simulink model "Pedal_Interpretation_exe"  (Simulink 7.0)
settings: Solver=ode4  StartTime=0.0  StopTime=88  FixedStep=0.01  RelTol=1e-3
InitFcn:
  | PedalInterp_para
values from neighbouring files (symbols this model uses):
  ped_min = 5    [PedalInterp_para.m]
  T_max_Brake = 4000    [PedalInterp_para.m]
  TI = 0    [PAS_callback.m]
undefined symbols (not defined in the file or in its folder): fzgbib, m_ab_100pro, m_ab_70pro, PedalInterpretation, v_bereich
libraries: simulink x320
(part 2 of 23)

== system Pedal_Interpretation_exe/TestData 1/SR-PI-02.2 Acceleration pedal interpretation/Initialisation & Stabilisation ==
  Constant 1 : Constant  Value=0  OutDataType=sfix(16)  OutScaling=2^0
  Constant 2 : Constant  Value=0  OutDataType=sfix(16)  OutScaling=2^0
  Constant 3 : Constant  Value=0  OutDataType=sfix(16)  OutScaling=2^0
  v_Fzg neutral : Outport  OutDataType=sfix(16)  OutScaling=2^0
  phi_Acc neutral : Outport  Port=2  OutDataType=sfix(16)  OutScaling=2^0
  phi_Brake neutral : Outport  Port=3  OutDataType=sfix(16)  OutScaling=2^0
  wires:
  Constant 1/1 -> v_Fzg neutral/1  "Constant 1"
  Constant 2/1 -> phi_Acc neutral/1  "Constant 2"
  Constant 3/1 -> phi_Brake neutral/1  "Constant 3"

== system Pedal_Interpretation_exe/TestData 1/SR-PI-02.2 Acceleration pedal interpretation/v = const & phi_Acc = const ==
  Generate constant 5 : Subsystem
  Generate constant 6 : Subsystem
  v_Fzg : Outport  OutDataType=sfix(16)  OutScaling=2^0
  phi_Acc : Outport  Port=2  OutDataType=sfix(16)  OutScaling=2^0
  wires:
  Generate constant 5/1(v_Fzg) -> v_Fzg/1
  Generate constant 6/1(phi_Acc) -> phi_Acc/1

== system Pedal_Interpretation_exe/TestData 1/SR-PI-02.2 Acceleration pedal interpretation/v = const & phi_Acc decreases & T_des_Drive < 0 ==
  Out Bus : Inport  OutDataType=sfix(16)  OutScaling=2^0
  <Constant>2 : Constant  Value=0  OutDataType=sfix(16)  OutScaling=2^0
  Bound Precond2 : Subsystem  mask(Bound){cm=<}
      mask prompts: cm "Comparison method:"
      mask help:
      | Compare a signal with a reference using the specified comparison method.
      |
      | For '==' or '~=' use "Range - Gap"
      mask init:
      | bp = get_param(gcbh,'Parent');
      | bn = get_param(gcbh,'Name');
      | set_param([bp '/' bn '/RelOp'],'Operator',get_param(gcbh,'cm'));
      mask StyleString: popup(>|>=|<=|<)
      mask Display:
      | port_label('output', 1, 'A');
      | port_label('input', 1, 'Sig');
      | port_label('input', 2, 'Ref');
      | text(0.05,0.5,get_param(get_param([get_param(gcb,'Parent') '/' get_param(gcb,'Name') '/RelOp'],'handle'),'Operator'));
  Bus Selector : BusSelector  OutputSignals=signal1.T_des_Drive
  Generate constant 6 : Subsystem
  Generate decrease 7 : Subsystem
  Memory T_des_Drive : Memory
  Activate : Outport  OutDataType=sfix(16)  OutScaling=2^0
  v_Fzg : Outport  Port=2  OutDataType=sfix(16)  OutScaling=2^0
  phi_Acc : Outport  Port=3  OutDataType=sfix(16)  OutScaling=2^0
  wires:
  Out Bus/1 -> Bus Selector/1
  Bus Selector/1 -> Memory T_des_Drive/1  "<T_des_Drive>"
  Memory T_des_Drive/1 -> Bound Precond2/1(Signal)
  <Constant>2/1 -> Bound Precond2/2(Reference)
  Bound Precond2/1(Activate) -> Activate/1
  Generate constant 6/1(v_Fzg) -> v_Fzg/1
  Generate decrease 7/1(phi_Acc) -> phi_Acc/1

== system Pedal_Interpretation_exe/TestData 1/SR-PI-02.2 Acceleration pedal interpretation/v = const & phi_Acc decreases & T_des_Drive >= 0 ==
  Out Bus : Inport  OutDataType=sfix(16)  OutScaling=2^0
  <Constant>2 : Constant  Value=0  OutDataType=sfix(16)  OutScaling=2^0
  Bound Precond2 : Subsystem  mask(Bound){cm=>=}
      mask prompts: cm "Comparison method:"
      mask help:
      | Compare a signal with a reference using the specified comparison method.
      |
      | For '==' or '~=' use "Range - Gap"
      mask init:
      | bp = get_param(gcbh,'Parent');
      | bn = get_param(gcbh,'Name');
      | set_param([bp '/' bn '/RelOp'],'Operator',get_param(gcbh,'cm'));
      mask StyleString: popup(>|>=|<=|<)
      mask Display:
      | port_label('output', 1, 'A');
      | port_label('input', 1, 'Sig');
      | port_label('input', 2, 'Ref');
      | text(0.05,0.5,get_param(get_param([get_param(gcb,'Parent') '/' get_param(gcb,'Name') '/RelOp'],'handle'),'Operator'));
  Bus Selector : BusSelector  OutputSignals=signal1.T_des_Drive
  Generate constant 6 : Subsystem
  Generate decrease 7 : Subsystem
  Memory T_des_Drive : Memory
  Activate : Outport  OutDataType=sfix(16)  OutScaling=2^0
  v_Fzg : Outport  Port=2  OutDataType=sfix(16)  OutScaling=2^0
  phi_Acc : Outport  Port=3  OutDataType=sfix(16)  OutScaling=2^0
  wires:
  Out Bus/1 -> Bus Selector/1
  Bus Selector/1 -> Memory T_des_Drive/1  "<T_des_Drive>"
  Memory T_des_Drive/1 -> Bound Precond2/1(Signal)
  <Constant>2/1 -> Bound Precond2/2(Reference)
  Bound Precond2/1(Activate) -> Activate/1
  Generate constant 6/1(v_Fzg) -> v_Fzg/1
  Generate decrease 7/1(phi_Acc) -> phi_Acc/1

== system Pedal_Interpretation_exe/TestData 1/SR-PI-02.2 Acceleration pedal interpretation/v = const & phi_Acc increases & T_des_Drive < 0 ==
  Out Bus : Inport  OutDataType=sfix(16)  OutScaling=2^0
  <Constant>2 : Constant  Value=0  OutDataType=sfix(16)  OutScaling=2^0
  Bound Precond2 : Subsystem  mask(Bound){cm=<}
      mask prompts: cm "Comparison method:"
      mask help:
      | Compare a signal with a reference using the specified comparison method.
      |
      | For '==' or '~=' use "Range - Gap"
      mask init:
      | bp = get_param(gcbh,'Parent');
      | bn = get_param(gcbh,'Name');
      | set_param([bp '/' bn '/RelOp'],'Operator',get_param(gcbh,'cm'));
      mask StyleString: popup(>|>=|<=|<)
      mask Display:
      | port_label('output', 1, 'A');
      | port_label('input', 1, 'Sig');
      | port_label('input', 2, 'Ref');
      | text(0.05,0.5,get_param(get_param([get_param(gcb,'Parent') '/' get_param(gcb,'Name') '/RelOp'],'handle'),'Operator'));
  Bus Selector : BusSelector  OutputSignals=signal1.T_des_Drive
  Generate constant 6 : Subsystem
  Generate increase 7 : Subsystem
  Memory T_des_Drive : Memory
  Activate : Outport  OutDataType=sfix(16)  OutScaling=2^0
  v_Fzg : Outport  Port=2  OutDataType=sfix(16)  OutScaling=2^0
  phi_Acc : Outport  Port=3  OutDataType=sfix(16)  OutScaling=2^0
  wires:
  Out Bus/1 -> Bus Selector/1
  Bus Selector/1 -> Memory T_des_Drive/1  "<T_des_Drive>"
  Memory T_des_Drive/1 -> Bound Precond2/1(Signal)
  <Constant>2/1 -> Bound Precond2/2(Reference)
  Bound Precond2/1(Activate) -> Activate/1
  Generate constant 6/1(v_Fzg) -> v_Fzg/1
  Generate increase 7/1(phi_Acc) -> phi_Acc/1

== system Pedal_Interpretation_exe/TestData 1/SR-PI-02.2 Acceleration pedal interpretation/v = const & phi_Acc increases & T_des_Drive >= 0 ==
  Out Bus : Inport  OutDataType=sfix(16)  OutScaling=2^0
  <Constant>2 : Constant  Value=0  OutDataType=sfix(16)  OutScaling=2^0
  Bound Precond2 : Subsystem  mask(Bound){cm=>=}
      mask prompts: cm "Comparison method:"
      mask help:
      | Compare a signal with a reference using the specified comparison method.
      |
      | For '==' or '~=' use "Range - Gap"
      mask init:
      | bp = get_param(gcbh,'Parent');
      | bn = get_param(gcbh,'Name');
      | set_param([bp '/' bn '/RelOp'],'Operator',get_param(gcbh,'cm'));
      mask StyleString: popup(>|>=|<=|<)
      mask Display:
      | port_label('output', 1, 'A');
      | port_label('input', 1, 'Sig');
      | port_label('input', 2, 'Ref');
      | text(0.05,0.5,get_param(get_param([get_param(gcb,'Parent') '/' get_param(gcb,'Name') '/RelOp'],'handle'),'Operator'));
  Bus Selector : BusSelector  OutputSignals=signal1.T_des_Drive
  Generate constant 6 : Subsystem
  Generate increase 7 : Subsystem
  Memory T_des_Drive : Memory
  Activate : Outport  OutDataType=sfix(16)  OutScaling=2^0
  v_Fzg : Outport  Port=2  OutDataType=sfix(16)  OutScaling=2^0
  phi_Acc : Outport  Port=3  OutDataType=sfix(16)  OutScaling=2^0
  wires:
  Out Bus/1 -> Bus Selector/1
  Bus Selector/1 -> Memory T_des_Drive/1  "<T_des_Drive>"
  Memory T_des_Drive/1 -> Bound Precond2/1(Signal)
  <Constant>2/1 -> Bound Precond2/2(Reference)
  Bound Precond2/1(Activate) -> Activate/1
  Generate constant 6/1(v_Fzg) -> v_Fzg/1
  Generate increase 7/1(phi_Acc) -> phi_Acc/1

== system Pedal_Interpretation_exe/TestData 1/SR-PI-02.2 Acceleration pedal interpretation/v increases & phi_Acc = const & T_des_Drive >= 0 ==
  Out Bus : Inport  OutDataType=sfix(16)  OutScaling=2^0
  <Constant>2 : Constant  Value=0  OutDataType=sfix(16)  OutScaling=2^0
  Bound Precond2 : Subsystem  mask(Bound){cm=>=}
      mask prompts: cm "Comparison method:"
      mask help:
      | Compare a signal with a reference using the specified comparison method.
      |
      | For '==' or '~=' use "Range - Gap"
      mask init:
      | bp = get_param(gcbh,'Parent');
      | bn = get_param(gcbh,'Name');
      | set_param([bp '/' bn '/RelOp'],'Operator',get_param(gcbh,'cm'));
      mask StyleString: popup(>|>=|<=|<)
      mask Display:
      | port_label('output', 1, 'A');
      | port_label('input', 1, 'Sig');
      | port_label('input', 2, 'Ref');
      | text(0.05,0.5,get_param(get_param([get_param(gcb,'Parent') '/' get_param(gcb,'Name') '/RelOp'],'handle'),'Operator'));
  Bus Selector : BusSelector  OutputSignals=signal1.T_des_Drive
  Generate constant 6 : Subsystem
  Generate increase 7 : Subsystem
  Memory T_des_Drive : Memory
  Activate : Outport  OutDataType=sfix(16)  OutScaling=2^0
  phi_Acc : Outport  Port=2  OutDataType=sfix(16)  OutScaling=2^0
  v_Fzg : Outport  Port=3  OutDataType=sfix(16)  OutScaling=2^0
  wires:
  Out Bus/1 -> Bus Selector/1
  Bus Selector/1 -> Memory T_des_Drive/1  "<T_des_Drive>"
  Memory T_des_Drive/1 -> Bound Precond2/1(Signal)
  <Constant>2/1 -> Bound Precond2/2(Reference)
  Bound Precond2/1(Activate) -> Activate/1
  Generate constant 6/1(phi_Acc) -> phi_Acc/1
  Generate increase 7/1(v_Fzg) -> v_Fzg/1

== system Pedal_Interpretation_exe/Validation Functions/SR-PI-01.1 Brake Pedal recognition/BrakePedal == 0 ==
  Activate : Inport  OutDataType=sfix(16)  OutScaling=2^0
  InOut Bus : Inport  Port=2  OutDataType=sfix(16)  OutScaling=2^0
  Bus Selector : BusSelector  OutputSignals=Outputs.signal2.BrakePedal
  Constant : Constant  Value=0  OutDataType=sfix(16)  OutScaling=2^0
  PAS : Subsystem  mask{AFT=TI, AFD=0}
      mask prompts: AFT "Assertion feature type:"; AFD "Assertion feature delay (in time steps)"
      mask init:
      | PAS_init(gcb);
      mask StyleString: popup(TI|TDD|TID),edit
      mask CallbackString: PAS_callback(gcb);|
  Range - Gap Relative tolerance Ass : Subsystem  mask(Range - Gap Relative Tolerance){GorR=Range, RelativeTolerance=0.0001}
      mask prompts: GorR "Use range or gap"; RelativeTolerance "Relative Tolerance in Percent"
      mask help: Check that a signal stays inside a range or outside a gap around a reference signal. Specify the range or the gap relative to the reference signal.
      mask init:
      | if max(get_param(gcb,'GorR') == ' ') % Gap
      |     helpVariable1 = '>=';
      |     helpVariable2 = '~=';
      | else % Range
      |     helpVariable1 = '<=';
      |     helpVariable2 = '==';
      | end
      | set_param([get_param(gcb,'Parent') '/' get_param(gcb,'Name') '/Relational Operator'],'Operator',helpVariable1);
      | clear helpVariable1;
      mask StyleString: popup(Range|Gap  ),edit
      mask Display:
      | port_label('output',1,'V');
      | port_label('input',1,'Sig');
      | port_label('input',2,'Ref');
      | text(0.35,0.5,[num2str(RelativeTolerance) '%']);
      | text(0.05,0.5,helpVariable2);
  VF info : Outport  OutDataType=sfix(16)  OutScaling=2^0
  wires:
  PAS/1(VF Info) -> VF info/1
  Bus Selector/1 -> Range - Gap Relative tolerance Ass/1(Signal)  "<BrakePedal>"
  Constant/1 -> Range - Gap Relative tolerance Ass/2(Reference)
  InOut Bus/1 -> Bus Selector/1
  Activate/1 -> PAS/1(Precond)
  Range - Gap Relative tolerance Ass/1(V) -> PAS/2(V)

== system Pedal_Interpretation_exe/Validation Functions/SR-PI-01.1 Brake Pedal recognition/BrakePedal == 1 ==
  Activate : Inport  OutDataType=sfix(16)  OutScaling=2^0
  InOut Bus : Inport  Port=2  OutDataType=sfix(16)  OutScaling=2^0
  Bus Selector : BusSelector  OutputSignals=Outputs.signal2.BrakePedal
  Constant : Constant  OutDataType=sfix(16)  OutScaling=2^0
  PAS : Subsystem  mask{AFT=TI, AFD=0}
      mask prompts: AFT "Assertion feature type:"; AFD "Assertion feature delay (in time steps)"
      mask init:
      | PAS_init(gcb);
      mask StyleString: popup(TI|TDD|TID),edit
      mask CallbackString: PAS_callback(gcb);|
  Range - Gap Relative tolerance Ass : Subsystem  mask(Range - Gap Relative Tolerance){GorR=Range, RelativeTolerance=0.0001}
      mask prompts: GorR "Use range or gap"; RelativeTolerance "Relative Tolerance in Percent"
      mask help: Check that a signal stays inside a range or outside a gap around a reference signal. Specify the range or the gap relative to the reference signal.
      mask init: same as Pedal_Interpretation_exe/Validation Functions/SR-PI-01.1 Brake Pedal recognition/BrakePedal == 0/Range - Gap Relative tolerance Ass
      mask StyleString: popup(Range|Gap  ),edit
      mask Display:
      | port_label('output',1,'V');
      | port_label('input',1,'Sig');
      | port_label('input',2,'Ref');
      | text(0.35,0.5,[num2str(RelativeTolerance) '%']);
      | text(0.05,0.5,helpVariable2);
  VF info : Outport  OutDataType=sfix(16)  OutScaling=2^0
  wires:
  PAS/1(VF Info) -> VF info/1
  Bus Selector/1 -> Range - Gap Relative tolerance Ass/1(Signal)  "<BrakePedal>"
  Constant/1 -> Range - Gap Relative tolerance Ass/2(Reference)
  InOut Bus/1 -> Bus Selector/1
  Activate/1 -> PAS/1(Precond)
  Range - Gap Relative tolerance Ass/1(V) -> PAS/2(V)

== system Pedal_Interpretation_exe/Validation Functions/SR-PI-01.1 Brake Pedal recognition/phi_Brake < ped_min ==
  InOut Bus : Inport  OutDataType=sfix(16)  OutScaling=2^0
  Bound Precond : Subsystem  mask(Bound){cm=<}
      mask prompts: cm "Comparison method:"
      mask help:
      | Compare a signal with a reference using the specified comparison method.
      |
      | For '==' or '~=' use "Range - Gap"
      mask init:
      | bp = get_param(gcbh,'Parent');
      | bn = get_param(gcbh,'Name');
      | set_param([bp '/' bn '/RelOp'],'Operator',get_param(gcbh,'cm'));
      mask StyleString: popup(>|>=|<=|<)
      mask Display:
      | port_label('output', 1, 'A');
      | port_label('input', 1, 'Sig');
      | port_label('input', 2, 'Ref');
      | text(0.05,0.5,get_param(get_param([get_param(gcb,'Parent') '/' get_param(gcb,'Name') '/RelOp'],'handle'),'Operator'));
  Bus Selector : BusSelector  OutputSignals=Inputs.signal2.phi_Brake
  Constant : Constant  Value=ped_min  OutDataType=sfix(16)  OutScaling=2^0
  PS : Subsystem  mask(Feature layer: preconditions synchronization){NoTI=1, NoTDD=0, NoTID=0, TIdel=[0], TDDdel=[]}
      mask prompts: NoTI "Time-independent features identifiable with or without a delay (TI)"; NoTDD "Triggered features identifiable with determinate delay or without a delay (TDD)"; NoTID "Triggered features identifiable with indeterminate delay (TID)"; TIdel "Time-independent features delays (in time steps). E.g. [0 1 0] for 3 features"; TDDdel "Triggered features delays (in time steps). E.g. [0 0] for 2 features"
      mask help: Use this block for synchronizing the precondition features. For changing the block inputs, use the parameters below. The output must be used for assertions activation.
      mask init:
      | PS_init(gcb);
      mask StyleString: popup(0|1|2|3|4|5|6|7|8|9),popup(0|1|2|3|4|5|6|7|8|9),popup(0|1|2|3|4|5|6|7|8|9),edit,edit
      mask CallbackString:
      | PSTI_callback(gcb);|PSTDD_callback(gcb);|PSTID_callback(gcb);|NoTI = str2double(get_param(gcb,'NoTI'));
      | TIdel = str2num(get_param(gcb,'TIdel'));
      | if NoTI ~= length(TIdel) && NoTI ~= 0
      |     error(['The number of delays entered (' num2str(length(TIdel)) ') does not correspond to the above specified number of time-independent features (' num2str(NoTI) ').']);
      | end|NoTDD = str2double(get_param(gcb,'NoTDD'));
      | TDDdel = str2num(get_param(gcb,'TDDdel'));
      | if NoTDD ~= length(TDDdel) && NoTDD ~= 0
      |     error(['The number of delays entered (' num2str(length(TDDdel)) ') does not correspond to the above specified number of triggered features with constant delay (' num2str(NoTDD) ').']);
      | end
  Activate : Outport  OutDataType=sfix(16)  OutScaling=2^0
  wires:
  InOut Bus/1 -> Bus Selector/1
  Bus Selector/1 -> Bound Precond/1(Signal)  "<phi_Brake>"
  Constant/1 -> Bound Precond/2(Reference)
  PS/1(Precond) -> Activate/1
  Bound Precond/1(Activate) -> PS/1(A TI1)

== system Pedal_Interpretation_exe/Validation Functions/SR-PI-01.1 Brake Pedal recognition/phi_Brake >= ped_min ==
  InOut Bus : Inport  OutDataType=sfix(16)  OutScaling=2^0
  Bound Precond : Subsystem  mask(Bound){cm=>=}
      mask prompts: cm "Comparison method:"
      mask help:
      | Compare a signal with a reference using the specified comparison method.
      |
      | For '==' or '~=' use "Range - Gap"
      mask init:
      | bp = get_param(gcbh,'Parent');
      | bn = get_param(gcbh,'Name');
      | set_param([bp '/' bn '/RelOp'],'Operator',get_param(gcbh,'cm'));
      mask StyleString: popup(>|>=|<=|<)
      mask Display:
      | port_label('output', 1, 'A');
      | port_label('input', 1, 'Sig');
      | port_label('input', 2, 'Ref');
      | text(0.05,0.5,get_param(get_param([get_param(gcb,'Parent') '/' get_param(gcb,'Name') '/RelOp'],'handle'),'Operator'));
  Bus Selector : BusSelector  OutputSignals=Inputs.signal2.phi_Brake
  Constant : Constant  Value=ped_min  OutDataType=sfix(16)  OutScaling=2^0
  PS : Subsystem  mask(Feature layer: preconditions synchronization){NoTI=1, NoTDD=0, NoTID=0, TIdel=[0], TDDdel=[]}
      mask prompts: NoTI "Time-independent features identifiable with or without a delay (TI)"; NoTDD "Triggered features identifiable with determinate delay or without a delay (TDD)"; NoTID "Triggered features identifiable with indeterminate delay (TID)"; TIdel "Time-independent features delays (in time steps). E.g. [0 1 0] for 3 features"; TDDdel "Triggered features delays (in time steps). E.g. [0 0] for 2 features"
      mask help: Use this block for synchronizing the precondition features. For changing the block inputs, use the parameters below. The output must be used for assertions activation.
      mask init:
      | PS_init(gcb);
      mask StyleString: popup(0|1|2|3|4|5|6|7|8|9),popup(0|1|2|3|4|5|6|7|8|9),popup(0|1|2|3|4|5|6|7|8|9),edit,edit
      mask CallbackString:
      | PSTI_callback(gcb);|PSTDD_callback(gcb);|PSTID_callback(gcb);|NoTI = str2double(get_param(gcb,'NoTI'));
      | TIdel = str2num(get_param(gcb,'TIdel'));
      | if NoTI ~= length(TIdel) && NoTI ~= 0
      |     error(['The number of delays entered (' num2str(length(TIdel)) ') does not correspond to the above specified number of time-independent features (' num2str(NoTI) ').']);
      | end|NoTDD = str2double(get_param(gcb,'NoTDD'));
      | TDDdel = str2num(get_param(gcb,'TDDdel'));
      | if NoTDD ~= length(TDDdel) && NoTDD ~= 0
      |     error(['The number of delays entered (' num2str(length(TDDdel)) ') does not correspond to the above specified number of triggered features with constant delay (' num2str(NoTDD) ').']);
      | end
  Activate : Outport  OutDataType=sfix(16)  OutScaling=2^0
  wires:
  InOut Bus/1 -> Bus Selector/1
  Bus Selector/1 -> Bound Precond/1(Signal)  "<phi_Brake>"
  PS/1(Precond) -> Activate/1
  Constant/1 -> Bound Precond/2(Reference)
  Bound Precond/1(Activate) -> PS/1(A TI1)

== system Pedal_Interpretation_exe/Validation Functions/SR-PI-01.3 Acceleration Pedal recognition/AccPedal == 0 ==
  Activate : Inport  OutDataType=sfix(16)  OutScaling=2^0
  InOut Bus : Inport  Port=2  OutDataType=sfix(16)  OutScaling=2^0
  Bus Selector : BusSelector  OutputSignals=Outputs.signal2.AccPedal
  Constant : Constant  Value=0  OutDataType=sfix(16)  OutScaling=2^0
  PAS : Subsystem  mask{AFT=TI, AFD=0}
      mask prompts: AFT "Assertion feature type:"; AFD "Assertion feature delay (in time steps)"
      mask init:
      | PAS_init(gcb);
      mask StyleString: popup(TI|TDD|TID),edit
      mask CallbackString: PAS_callback(gcb);|
  Range - Gap Relative tolerance Ass : Subsystem  mask(Range - Gap Relative Tolerance){GorR=Range, RelativeTolerance=0.0001}
      mask prompts: GorR "Use range or gap"; RelativeTolerance "Relative Tolerance in Percent"
      mask help: Check that a signal stays inside a range or outside a gap around a reference signal. Specify the range or the gap relative to the reference signal.
      mask init: same as Pedal_Interpretation_exe/Validation Functions/SR-PI-01.1 Brake Pedal recognition/BrakePedal == 0/Range - Gap Relative tolerance Ass
      mask StyleString: popup(Range|Gap  ),edit
      mask Display:
      | port_label('output',1,'V');
      | port_label('input',1,'Sig');
      | port_label('input',2,'Ref');
      | text(0.35,0.5,[num2str(RelativeTolerance) '%']);
      | text(0.05,0.5,helpVariable2);
  VF info : Outport  OutDataType=sfix(16)  OutScaling=2^0
  wires:
  InOut Bus/1 -> Bus Selector/1
  Bus Selector/1 -> Range - Gap Relative tolerance Ass/1(Signal)  "<AccPedal>"
  Constant/1 -> Range - Gap Relative tolerance Ass/2(Reference)
  PAS/1(VF Info) -> VF info/1
  Activate/1 -> PAS/1(Precond)
  Range - Gap Relative tolerance Ass/1(V) -> PAS/2(V)

== system Pedal_Interpretation_exe/Validation Functions/SR-PI-01.3 Acceleration Pedal recognition/AccPedal == 1 ==
  Activate : Inport  OutDataType=sfix(16)  OutScaling=2^0
  InOut Bus : Inport  Port=2  OutDataType=sfix(16)  OutScaling=2^0
  Bus Selector : BusSelector  OutputSignals=Outputs.signal2.AccPedal
  Constant : Constant  OutDataType=sfix(16)  OutScaling=2^0
  PAS : Subsystem  mask{AFT=TI, AFD=0}
      mask prompts: AFT "Assertion feature type:"; AFD "Assertion feature delay (in time steps)"
      mask init:
      | PAS_init(gcb);
      mask StyleString: popup(TI|TDD|TID),edit
      mask CallbackString: PAS_callback(gcb);|
  Range - Gap Relative tolerance Ass : Subsystem  mask(Range - Gap Relative Tolerance){GorR=Range, RelativeTolerance=0.0001}
      mask prompts: GorR "Use range or gap"; RelativeTolerance "Relative Tolerance in Percent"
      mask help: Check that a signal stays inside a range or outside a gap around a reference signal. Specify the range or the gap relative to the reference signal.
      mask init: same as Pedal_Interpretation_exe/Validation Functions/SR-PI-01.1 Brake Pedal recognition/BrakePedal == 0/Range - Gap Relative tolerance Ass
      mask StyleString: popup(Range|Gap  ),edit
      mask Display:
      | port_label('output',1,'V');
      | port_label('input',1,'Sig');
      | port_label('input',2,'Ref');
      | text(0.35,0.5,[num2str(RelativeTolerance) '%']);
      | text(0.05,0.5,helpVariable2);
  VF info : Outport  OutDataType=sfix(16)  OutScaling=2^0
  wires:
  InOut Bus/1 -> Bus Selector/1
  PAS/1(VF Info) -> VF info/1
  Bus Selector/1 -> Range - Gap Relative tolerance Ass/1(Signal)  "<AccPedal>"
  Constant/1 -> Range - Gap Relative tolerance Ass/2(Reference)
  Activate/1 -> PAS/1(Precond)
  Range - Gap Relative tolerance Ass/1(V) -> PAS/2(V)

== system Pedal_Interpretation_exe/Validation Functions/SR-PI-01.3 Acceleration Pedal recognition/phi_Acc < ped_min ==
  InOut Bus : Inport  OutDataType=sfix(16)  OutScaling=2^0
  Bound Precond : Subsystem  mask(Bound){cm=<}
      mask prompts: cm "Comparison method:"
      mask help:
      | Compare a signal with a reference using the specified comparison method.
      |
      | For '==' or '~=' use "Range - Gap"
      mask init:
      | bp = get_param(gcbh,'Parent');
      | bn = get_param(gcbh,'Name');
      | set_param([bp '/' bn '/RelOp'],'Operator',get_param(gcbh,'cm'));
      mask StyleString: popup(>|>=|<=|<)
      mask Display:
      | port_label('output', 1, 'A');
      | port_label('input', 1, 'Sig');
      | port_label('input', 2, 'Ref');
      | text(0.05,0.5,get_param(get_param([get_param(gcb,'Parent') '/' get_param(gcb,'Name') '/RelOp'],'handle'),'Operator'));
  Bus Selector : BusSelector  OutputSignals=Inputs.signal2.phi_Acc
  Constant : Constant  Value=ped_min  OutDataType=sfix(16)  OutScaling=2^0
  PS : Subsystem  mask(Feature layer: preconditions synchronization){NoTI=1, NoTDD=0, NoTID=0, TIdel=[0], TDDdel=[]}
      mask prompts: NoTI "Time-independent features identifiable with or without a delay (TI)"; NoTDD "Triggered features identifiable with determinate delay or without a delay (TDD)"; NoTID "Triggered features identifiable with indeterminate delay (TID)"; TIdel "Time-independent features delays (in time steps). E.g. [0 1 0] for 3 features"; TDDdel "Triggered features delays (in time steps). E.g. [0 0] for 2 features"
      mask help: Use this block for synchronizing the precondition features. For changing the block inputs, use the parameters below. The output must be used for assertions activation.
      mask init:
      | PS_init(gcb);
      mask StyleString: popup(0|1|2|3|4|5|6|7|8|9),popup(0|1|2|3|4|5|6|7|8|9),popup(0|1|2|3|4|5|6|7|8|9),edit,edit
      mask CallbackString:
      | PSTI_callback(gcb);|PSTDD_callback(gcb);|PSTID_callback(gcb);|NoTI = str2double(get_param(gcb,'NoTI'));
      | TIdel = str2num(get_param(gcb,'TIdel'));
      | if NoTI ~= length(TIdel) && NoTI ~= 0
      |     error(['The number of delays entered (' num2str(length(TIdel)) ') does not correspond to the above specified number of time-independent features (' num2str(NoTI) ').']);
      | end|NoTDD = str2double(get_param(gcb,'NoTDD'));
      | TDDdel = str2num(get_param(gcb,'TDDdel'));
      | if NoTDD ~= length(TDDdel) && NoTDD ~= 0
      |     error(['The number of delays entered (' num2str(length(TDDdel)) ') does not correspond to the above specified number of triggered features with constant delay (' num2str(NoTDD) ').']);
      | end
  Activate : Outport  OutDataType=sfix(16)  OutScaling=2^0
  wires:
  InOut Bus/1 -> Bus Selector/1
  Bus Selector/1 -> Bound Precond/1(Signal)  "<phi_Acc>"
  Constant/1 -> Bound Precond/2(Reference)
  Bound Precond/1(Activate) -> PS/1(A TI1)
  PS/1(Precond) -> Activate/1

== system Pedal_Interpretation_exe/Validation Functions/SR-PI-01.3 Acceleration Pedal recognition/phi_Acc >= ped_min ==
  InOut Bus : Inport  OutDataType=sfix(16)  OutScaling=2^0
  Bound Precond : Subsystem  mask(Bound){cm=>=}
      mask prompts: cm "Comparison method:"
      mask help:
      | Compare a signal with a reference using the specified comparison method.
      |
      | For '==' or '~=' use "Range - Gap"
      mask init:
      | bp = get_param(gcbh,'Parent');
      | bn = get_param(gcbh,'Name');
      | set_param([bp '/' bn '/RelOp'],'Operator',get_param(gcbh,'cm'));
      mask StyleString: popup(>|>=|<=|<)
      mask Display:
      | port_label('output', 1, 'A');
      | port_label('input', 1, 'Sig');
      | port_label('input', 2, 'Ref');
      | text(0.05,0.5,get_param(get_param([get_param(gcb,'Parent') '/' get_param(gcb,'Name') '/RelOp'],'handle'),'Operator'));
  Bus Selector : BusSelector  OutputSignals=Inputs.signal2.phi_Acc
  Constant : Constant  Value=ped_min  OutDataType=sfix(16)  OutScaling=2^0
  PS : Subsystem  mask(Feature layer: preconditions synchronization){NoTI=1, NoTDD=0, NoTID=0, TIdel=[0], TDDdel=[]}
      mask prompts: NoTI "Time-independent features identifiable with or without a delay (TI)"; NoTDD "Triggered features identifiable with determinate delay or without a delay (TDD)"; NoTID "Triggered features identifiable with indeterminate delay (TID)"; TIdel "Time-independent features delays (in time steps). E.g. [0 1 0] for 3 features"; TDDdel "Triggered features delays (in time steps). E.g. [0 0] for 2 features"
      mask help: Use this block for synchronizing the precondition features. For changing the block inputs, use the parameters below. The output must be used for assertions activation.
      mask init:
      | PS_init(gcb);
      mask StyleString: popup(0|1|2|3|4|5|6|7|8|9),popup(0|1|2|3|4|5|6|7|8|9),popup(0|1|2|3|4|5|6|7|8|9),edit,edit
      mask CallbackString:
      | PSTI_callback(gcb);|PSTDD_callback(gcb);|PSTID_callback(gcb);|NoTI = str2double(get_param(gcb,'NoTI'));
      | TIdel = str2num(get_param(gcb,'TIdel'));
      | if NoTI ~= length(TIdel) && NoTI ~= 0
      |     error(['The number of delays entered (' num2str(length(TIdel)) ') does not correspond to the above specified number of time-independent features (' num2str(NoTI) ').']);
      | end|NoTDD = str2double(get_param(gcb,'NoTDD'));
      | TDDdel = str2num(get_param(gcb,'TDDdel'));
      | if NoTDD ~= length(TDDdel) && NoTDD ~= 0
      |     error(['The number of delays entered (' num2str(length(TDDdel)) ') does not correspond to the above specified number of triggered features with constant delay (' num2str(NoTDD) ').']);
      | end
  Activate : Outport  OutDataType=sfix(16)  OutScaling=2^0
  wires:
  InOut Bus/1 -> Bus Selector/1
  Bus Selector/1 -> Bound Precond/1(Signal)  "<phi_Acc>"
  Constant/1 -> Bound Precond/2(Reference)
  PS/1(Precond) -> Activate/1
  Bound Precond/1(Activate) -> PS/1(A TI1)

== system Pedal_Interpretation_exe/Validation Functions/SR-PI-02.1 Brake pedal interpretation/phi_Brake/100 = T_des_Brake/T_max_Brake ==
  Activate : Inport  OutDataType=sfix(16)  OutScaling=2^0
  InOut Bus : Inport  Port=2  OutDataType=sfix(16)  OutScaling=2^0
  Bus Selector : BusSelector  OutputSignals=Outputs.signal1.T_des_Brake,Inputs.signal2.phi_Brake
  Constant : Constant  Value=T_max_Brake  OutDataType=sfix(16)  OutScaling=2^0
  Constant1 : Constant  Value=100  OutDataType=sfix(16)  OutScaling=2^0
  Divide : Product  Inputs=/*  OutDataType=sfix(16)  OutScaling=2^-10
  Divide1 : Product  Inputs=*/  OutDataType=sfix(16)  OutScaling=2^-10
  PAS : Subsystem  mask{AFT=TI, AFD=0}
      mask prompts: AFT "Assertion feature type:"; AFD "Assertion feature delay (in time steps)"
      mask init:
      | PAS_init(gcb);
      mask StyleString: popup(TI|TDD|TID),edit
      mask CallbackString: PAS_callback(gcb);|
  Range - Gap Relative tolerance Ass : Subsystem  mask(Range - Gap Relative Tolerance){GorR=Range, RelativeTolerance=0.0001}
      mask prompts: GorR "Use range or gap"; RelativeTolerance "Relative Tolerance in Percent"
      mask help: Check that a signal stays inside a range or outside a gap around a reference signal. Specify the range or the gap relative to the reference signal.
      mask init: same as Pedal_Interpretation_exe/Validation Functions/SR-PI-01.1 Brake Pedal recognition/BrakePedal == 0/Range - Gap Relative tolerance Ass
      mask StyleString: popup(Range|Gap  ),edit
      mask Display:
      | port_label('output',1,'V');
      | port_label('input',1,'Sig');
      | port_label('input',2,'Ref');
      | text(0.35,0.5,[num2str(RelativeTolerance) '%']);
      | text(0.05,0.5,helpVariable2);
  VF info : Outport  OutDataType=sfix(16)  OutScaling=2^0
  wires:
  InOut Bus/1 -> Bus Selector/1
  Divide/1 -> Range - Gap Relative tolerance Ass/1(Signal)
  Bus Selector/2 -> Divide1/1  "<phi_Brake>"
  Bus Selector/1 -> Divide/2  "<T_des_Brake>"
  Constant/1 -> Divide/1
  Constant1/1 -> Divide1/2
  PAS/1(VF Info) -> VF info/1
  Activate/1 -> PAS/1(Precond)
  Range - Gap Relative tolerance Ass/1(V) -> PAS/2(V)
  Divide1/1 -> Range - Gap Relative tolerance Ass/2(Reference)

== system Pedal_Interpretation_exe/Validation Functions/SR-PI-02.1 Brake pedal interpretation/true ==
  InOut Bus : Inport  OutDataType=sfix(16)  OutScaling=2^0
  Always active : Constant  OutDataType=sfix(16)  OutScaling=2^0
  PS : Subsystem  mask(Feature layer: preconditions synchronization){NoTI=1, NoTDD=0, NoTID=0, TIdel=[0], TDDdel=[]}
      mask prompts: NoTI "Time-independent features identifiable with or without a delay (TI)"; NoTDD "Triggered features identifiable with determinate delay or without a delay (TDD)"; NoTID "Triggered features identifiable with indeterminate delay (TID)"; TIdel "Time-independent features delays (in time steps). E.g. [0 1 0] for 3 features"; TDDdel "Triggered features delays (in time steps). E.g. [0 0] for 2 features"
      mask help: Use this block for synchronizing the precondition features. For changing the block inputs, use the parameters below. The output must be used for assertions activation.
      mask init:
      | PS_init(gcb);
      mask StyleString: popup(0|1|2|3|4|5|6|7|8|9),popup(0|1|2|3|4|5|6|7|8|9),popup(0|1|2|3|4|5|6|7|8|9),edit,edit
      mask CallbackString:
      | PSTI_callback(gcb);|PSTDD_callback(gcb);|PSTID_callback(gcb);|NoTI = str2double(get_param(gcb,'NoTI'));
      | TIdel = str2num(get_param(gcb,'TIdel'));
      | if NoTI ~= length(TIdel) && NoTI ~= 0
      |     error(['The number of delays entered (' num2str(length(TIdel)) ') does not correspond to the above specified number of time-independent features (' num2str(NoTI) ').']);
      | end|NoTDD = str2double(get_param(gcb,'NoTDD'));
      | TDDdel = str2num(get_param(gcb,'TDDdel'));
      | if NoTDD ~= length(TDDdel) && NoTDD ~= 0
      |     error(['The number of delays entered (' num2str(length(TDDdel)) ') does not correspond to the above specified number of triggered features with constant delay (' num2str(NoTDD) ').']);
      | end
  Terminator_1 : Terminator
  Activate : Outport  OutDataType=sfix(16)  OutScaling=2^0
  wires:
  InOut Bus/1 -> Terminator_1/1
  Always active/1 -> PS/1(A TI1)
  PS/1(Precond) -> Activate/1

== system Pedal_Interpretation_exe/Validation Functions/SR-PI-02.2 Acceleration pedal interpretation/T_des_Drive = const ==
  Activate : Inport  OutDataType=sfix(16)  OutScaling=2^0
  InOut Bus : Inport  Port=2  OutDataType=sfix(16)  OutScaling=2^0
  Bus Selector : BusSelector  OutputSignals=Outputs.signal1.T_des_Drive
  Constant : Constant  OutDataType=sfix(16)  OutScaling=2^0
  Detect constant : Subsystem  TreatAsAtomicUnit=on  mask(Feature extraction block){RT=1}
      mask prompts: RT "Relative tolerance in %"
      mask help: Detect if the signal value is constant (using the last two signal values) allowing for a user-defined relative deviation
      mask CallbackString:
      | if or( (str2double(get_param(gcb,'RT')) < 0), (str2double(get_param(gcb,'RT')) > 100))
      |     error(['Relative tolerance value (' get_param(gcb,'RT') ') out of range. Please give a value between 0 and 100.']);
      | else
      |     set_param([gcb '/Relative tolerance/Relative Tolerance'],'Value',get_param(gcb,'RT'));
      | end
  PAS : Subsystem  mask{AFT=TI, AFD=2}
      mask prompts: AFT "Assertion feature type:"; AFD "Assertion feature delay (in time steps)"
      mask init:
      | PAS_init(gcb);
      mask StyleString: popup(TI|TDD|TID),edit
      mask CallbackString: PAS_callback(gcb);|
  Range - Gap Relative tolerance Ass : Subsystem  mask(Range - Gap Relative Tolerance){GorR=Range, RelativeTolerance=0}
      mask prompts: GorR "Use range or gap"; RelativeTolerance "Relative Tolerance in Percent"
      mask help: Check that a signal stays inside a range or outside a gap around a reference signal. Specify the range or the gap relative to the reference signal.
      mask init: same as Pedal_Interpretation_exe/Validation Functions/SR-PI-01.1 Brake Pedal recognition/BrakePedal == 0/Range - Gap Relative tolerance Ass
      mask StyleString: popup(Range|Gap  ),edit
      mask Display:
      | port_label('output',1,'V');
      | port_label('input',1,'Sig');
      | port_label('input',2,'Ref');
      | text(0.35,0.5,[num2str(RelativeTolerance) '%']);
      | text(0.05,0.5,helpVariable2);
  VF info : Outport  OutDataType=sfix(16)  OutScaling=2^0
  wires:
  InOut Bus/1 -> Bus Selector/1
  Bus Selector/1 -> Detect constant/1(Signal)  "<T_des_Drive>"
  PAS/1(VF Info) -> VF info/1
  Activate/1 -> PAS/1(Precond)
  Constant/1 -> Range - Gap Relative tolerance Ass/2(Reference)
  Detect constant/1(Constant) -> Range - Gap Relative tolerance Ass/1(Signal)
  Range - Gap Relative tolerance Ass/1(V) -> PAS/2(V)

== system Pedal_Interpretation_exe/Validation Functions/SR-PI-02.2 Acceleration pedal interpretation/T_des_Drive decreases ==
  Activate : Inport  OutDataType=sfix(16)  OutScaling=2^0
  InOut Bus : Inport  Port=2  OutDataType=sfix(16)  OutScaling=2^0
  Bus Selector : BusSelector  OutputSignals=Outputs.signal1.T_des_Drive
  Constant : Constant  OutDataType=sfix(16)  OutScaling=2^0
  Detect decrease : Subsystem  TreatAsAtomicUnit=on  mask(Detect increase){Param=0}
      mask prompts: Param "Mask Parameter 1:"
  PAS : Subsystem  mask{AFT=TI, AFD=2}
      mask prompts: AFT "Assertion feature type:"; AFD "Assertion feature delay (in time steps)"
      mask init:
      | PAS_init(gcb);
      mask StyleString: popup(TI|TDD|TID),edit
      mask CallbackString: PAS_callback(gcb);|
  Range - Gap Relative tolerance Ass : Subsystem  mask(Range - Gap Relative Tolerance){GorR=Range, RelativeTolerance=0}
      mask prompts: GorR "Use range or gap"; RelativeTolerance "Relative Tolerance in Percent"
      mask help: Check that a signal stays inside a range or outside a gap around a reference signal. Specify the range or the gap relative to the reference signal.
      mask init: same as Pedal_Interpretation_exe/Validation Functions/SR-PI-01.1 Brake Pedal recognition/BrakePedal == 0/Range - Gap Relative tolerance Ass
      mask StyleString: popup(Range|Gap  ),edit
      mask Display:
      | port_label('output',1,'V');
      | port_label('input',1,'Sig');
      | port_label('input',2,'Ref');
      | text(0.35,0.5,[num2str(RelativeTolerance) '%']);
      | text(0.05,0.5,helpVariable2);
  VF info : Outport  OutDataType=sfix(16)  OutScaling=2^0
  wires:
  InOut Bus/1 -> Bus Selector/1
  Bus Selector/1 -> Detect decrease/1(Signal)  "<T_des_Drive>"
  Activate/1 -> PAS/1(Precond)
  PAS/1(VF Info) -> VF info/1
  Constant/1 -> Range - Gap Relative tolerance Ass/2(Reference)
  Detect decrease/1(Decrease) -> Range - Gap Relative tolerance Ass/1(Signal)
  Range - Gap Relative tolerance Ass/1(V) -> PAS/2(V)

== system Pedal_Interpretation_exe/Validation Functions/SR-PI-02.2 Acceleration pedal interpretation/T_des_Drive decreases  ==
  Activate : Inport  OutDataType=sfix(16)  OutScaling=2^0
  InOut Bus : Inport  Port=2  OutDataType=sfix(16)  OutScaling=2^0
  Bus Selector : BusSelector  OutputSignals=Outputs.signal1.T_des_Drive
  Constant : Constant  OutDataType=sfix(16)  OutScaling=2^0
  Detect decrease : Subsystem  TreatAsAtomicUnit=on  mask(Detect increase){Param=0}
      mask prompts: Param "Mask Parameter 1:"
  PAS : Subsystem  mask{AFT=TI, AFD=2}
      mask prompts: AFT "Assertion feature type:"; AFD "Assertion feature delay (in time steps)"
      mask init:
      | PAS_init(gcb);
      mask StyleString: popup(TI|TDD|TID),edit
      mask CallbackString: PAS_callback(gcb);|
  Range - Gap Relative tolerance Ass : Subsystem  mask(Range - Gap Relative Tolerance){GorR=Range, RelativeTolerance=0}
      mask prompts: GorR "Use range or gap"; RelativeTolerance "Relative Tolerance in Percent"
      mask help: Check that a signal stays inside a range or outside a gap around a reference signal. Specify the range or the gap relative to the reference signal.
      mask init: same as Pedal_Interpretation_exe/Validation Functions/SR-PI-01.1 Brake Pedal recognition/BrakePedal == 0/Range - Gap Relative tolerance Ass
      mask StyleString: popup(Range|Gap  ),edit
      mask Display:
      | port_label('output',1,'V');
      | port_label('input',1,'Sig');
      | port_label('input',2,'Ref');
      | text(0.35,0.5,[num2str(RelativeTolerance) '%']);
      | text(0.05,0.5,helpVariable2);
  VF info : Outport  OutDataType=sfix(16)  OutScaling=2^0
  wires:
  InOut Bus/1 -> Bus Selector/1
  Bus Selector/1 -> Detect decrease/1(Signal)  "<T_des_Drive>"
  PAS/1(VF Info) -> VF info/1
  Activate/1 -> PAS/1(Precond)
  Constant/1 -> Range - Gap Relative tolerance Ass/2(Reference)
  Detect decrease/1(Decrease) -> Range - Gap Relative tolerance Ass/1(Signal)
  Range - Gap Relative tolerance Ass/1(V) -> PAS/2(V)

== system Pedal_Interpretation_exe/Validation Functions/SR-PI-02.2 Acceleration pedal interpretation/T_des_Drive does not increase ==
  Activate : Inport  OutDataType=sfix(16)  OutScaling=2^0
  InOut Bus : Inport  Port=2  OutDataType=sfix(16)  OutScaling=2^0
  Bus Selector : BusSelector  OutputSignals=Outputs.signal1.T_des_Drive
  Constant : Constant  OutDataType=sfix(16)  OutScaling=2^0
  Detect 'does not increase' : Subsystem  TreatAsAtomicUnit=on  mask(Detect increase){Param=0}
      mask prompts: Param "Mask Parameter 1:"
  PAS : Subsystem  mask{AFT=TI, AFD=2}
      mask prompts: AFT "Assertion feature type:"; AFD "Assertion feature delay (in time steps)"
      mask init:
      | PAS_init(gcb);
      mask StyleString: popup(TI|TDD|TID),edit
      mask CallbackString: PAS_callback(gcb);|
  Range - Gap Relative tolerance Ass : Subsystem  mask(Range - Gap Relative Tolerance){GorR=Range, RelativeTolerance=0}
      mask prompts: GorR "Use range or gap"; RelativeTolerance "Relative Tolerance in Percent"
      mask help: Check that a signal stays inside a range or outside a gap around a reference signal. Specify the range or the gap relative to the reference signal.
      mask init: same as Pedal_Interpretation_exe/Validation Functions/SR-PI-01.1 Brake Pedal recognition/BrakePedal == 0/Range - Gap Relative tolerance Ass
      mask StyleString: popup(Range|Gap  ),edit
      mask Display:
      | port_label('output',1,'V');
      | port_label('input',1,'Sig');
      | port_label('input',2,'Ref');
      | text(0.35,0.5,[num2str(RelativeTolerance) '%']);
      | text(0.05,0.5,helpVariable2);
  VF info : Outport  OutDataType=sfix(16)  OutScaling=2^0
  wires:
  Bus Selector/1 -> Detect 'does not increase'/1(Signal)  "<T_des_Drive>"
  InOut Bus/1 -> Bus Selector/1
  Activate/1 -> PAS/1(Precond)
  PAS/1(VF Info) -> VF info/1
  Detect 'does not increase'/1(Decrease) -> Range - Gap Relative tolerance Ass/1(Signal)
  Constant/1 -> Range - Gap Relative tolerance Ass/2(Reference)
  Range - Gap Relative tolerance Ass/1(V) -> PAS/2(V)

== system Pedal_Interpretation_exe/Validation Functions/SR-PI-02.2 Acceleration pedal interpretation/T_des_Drive increases ==
  Activate : Inport  OutDataType=sfix(16)  OutScaling=2^0
  InOut Bus : Inport  Port=2  OutDataType=sfix(16)  OutScaling=2^0
  Bus Selector : BusSelector  OutputSignals=Outputs.signal1.T_des_Drive
  Constant : Constant  OutDataType=sfix(16)  OutScaling=2^0
  Detect increase : Subsystem  TreatAsAtomicUnit=on  mask(Detect increase){Param=0}
      mask prompts: Param "Mask Parameter 1:"
  PAS : Subsystem  mask{AFT=TI, AFD=2}
      mask prompts: AFT "Assertion feature type:"; AFD "Assertion feature delay (in time steps)"
      mask init:
      | PAS_init(gcb);
      mask StyleString: popup(TI|TDD|TID),edit
      mask CallbackString: PAS_callback(gcb);|
  Range - Gap Relative tolerance Ass : Subsystem  mask(Range - Gap Relative Tolerance){GorR=Range, RelativeTolerance=0}
      mask prompts: GorR "Use range or gap"; RelativeTolerance "Relative Tolerance in Percent"
      mask help: Check that a signal stays inside a range or outside a gap around a reference signal. Specify the range or the gap relative to the reference signal.
      mask init: same as Pedal_Interpretation_exe/Validation Functions/SR-PI-01.1 Brake Pedal recognition/BrakePedal == 0/Range - Gap Relative tolerance Ass
      mask StyleString: popup(Range|Gap  ),edit
      mask Display:
      | port_label('output',1,'V');
      | port_label('input',1,'Sig');
      | port_label('input',2,'Ref');
      | text(0.35,0.5,[num2str(RelativeTolerance) '%']);
      | text(0.05,0.5,helpVariable2);
  VF info : Outport  OutDataType=sfix(16)  OutScaling=2^0
  wires:
  InOut Bus/1 -> Bus Selector/1
  Bus Selector/1 -> Detect increase/1(Signal)  "<T_des_Drive>"
  PAS/1(VF Info) -> VF info/1
  Activate/1 -> PAS/1(Precond)
  Constant/1 -> Range - Gap Relative tolerance Ass/2(Reference)
  Detect increase/1(Increase) -> Range - Gap Relative tolerance Ass/1(Signal)
  Range - Gap Relative tolerance Ass/1(V) -> PAS/2(V)

== system Pedal_Interpretation_exe/Validation Functions/SR-PI-02.2 Acceleration pedal interpretation/T_des_Drive increases  ==
  Activate : Inport  OutDataType=sfix(16)  OutScaling=2^0
  InOut Bus : Inport  Port=2  OutDataType=sfix(16)  OutScaling=2^0
  Bus Selector : BusSelector  OutputSignals=Outputs.signal1.T_des_Drive
  Constant : Constant  OutDataType=sfix(16)  OutScaling=2^0
  Detect increase : Subsystem  TreatAsAtomicUnit=on  mask(Detect increase){Param=0}
      mask prompts: Param "Mask Parameter 1:"
  PAS : Subsystem  mask{AFT=TI, AFD=2}
      mask prompts: AFT "Assertion feature type:"; AFD "Assertion feature delay (in time steps)"
      mask init:
      | PAS_init(gcb);
      mask StyleString: popup(TI|TDD|TID),edit
      mask CallbackString: PAS_callback(gcb);|
  Range - Gap Relative tolerance Ass : Subsystem  mask(Range - Gap Relative Tolerance){GorR=Range, RelativeTolerance=0}
      mask prompts: GorR "Use range or gap"; RelativeTolerance "Relative Tolerance in Percent"
      mask help: Check that a signal stays inside a range or outside a gap around a reference signal. Specify the range or the gap relative to the reference signal.
      mask init: same as Pedal_Interpretation_exe/Validation Functions/SR-PI-01.1 Brake Pedal recognition/BrakePedal == 0/Range - Gap Relative tolerance Ass
      mask StyleString: popup(Range|Gap  ),edit
      mask Display:
      | port_label('output',1,'V');
      | port_label('input',1,'Sig');
      | port_label('input',2,'Ref');
      | text(0.35,0.5,[num2str(RelativeTolerance) '%']);
      | text(0.05,0.5,helpVariable2);
  VF info : Outport  OutDataType=sfix(16)  OutScaling=2^0
  wires:
  InOut Bus/1 -> Bus Selector/1
  Bus Selector/1 -> Detect increase/1(Signal)  "<T_des_Drive>"
  Activate/1 -> PAS/1(Precond)
  PAS/1(VF Info) -> VF info/1
  Constant/1 -> Range - Gap Relative tolerance Ass/2(Reference)
  Detect increase/1(Increase) -> Range - Gap Relative tolerance Ass/1(Signal)
  Range - Gap Relative tolerance Ass/1(V) -> PAS/2(V)
